simulink model "stage1_robust_loop_model"  (R2026a)
settings: Solver=ode45  StopTime=0.8
undefined symbols (not defined in the file): B, CPR, Ke, Kt, L, R, Ts_disc, V_dc
settings Model: Creator=knavn  LastModifiedBy=knavn

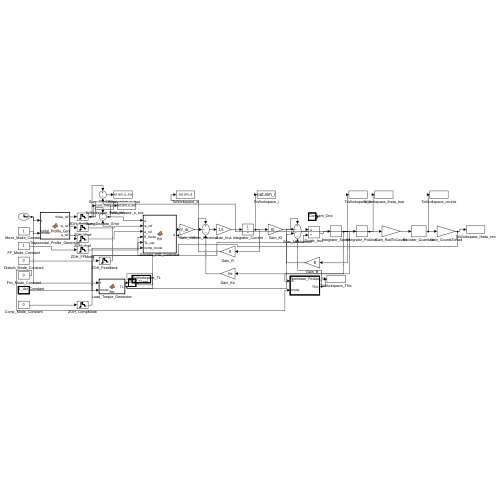
[thumbnail: Simulink's stored preview of the top-level diagram]
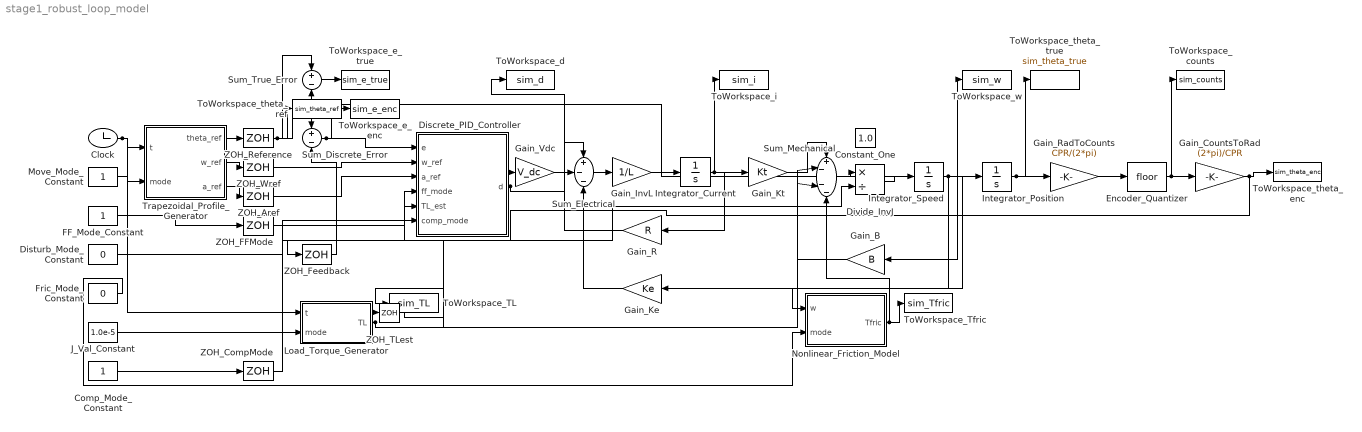
== system stage1_robust_loop_model ==
  Clock : Clock
  Comp_Mode_Constant : Constant
  Constant_One : Constant  Value=1.0
  Discrete_PID_Controller : MATLAB Function  TreatAsAtomicUnit=on
  Disturb_Mode_Constant : Constant  Value=0
  Divide_InvJ : Product  Inputs=*/
  Encoder_Quantizer : Rounding
  FF_Mode_Constant : Constant
  Fric_Mode_Constant : Constant  Value=0
  Gain_B : Gain  Gain=B
  Gain_CountsToRad : Gain  Gain=(2*pi)/CPR
  Gain_InvL : Gain  Gain=1/L
  Gain_Ke : Gain  Gain=Ke
  Gain_Kt : Gain  Gain=Kt
  Gain_R : Gain  Gain=R
  Gain_RadToCounts : Gain  Gain=CPR/(2*pi)
  Gain_Vdc : Gain  Gain=V_dc
  Integrator_Current : Integrator
  Integrator_Position : Integrator
  Integrator_Speed : Integrator
  J_Val_Constant : Constant  Value=1.0e-5
  Load_Torque_Generator : MATLAB Function  TreatAsAtomicUnit=on
  Move_Mode_Constant : Constant
  Nonlinear_Friction_Model : MATLAB Function  TreatAsAtomicUnit=on
  Sum_Discrete_Error : Sum  Inputs=+-
  Sum_Electrical : Sum  Inputs=+--
  Sum_Mechanical : Sum  Inputs=+---
  Sum_True_Error : Sum  Inputs=+-
  ToWorkspace_TL : ToWorkspace  VariableName=sim_TL  SaveFormat=Timeseries  SampleTime=-1
  ToWorkspace_Tfric : ToWorkspace  VariableName=sim_Tfric  SaveFormat=Timeseries  SampleTime=-1
  ToWorkspace_counts : ToWorkspace  VariableName=sim_counts  SaveFormat=Timeseries  SampleTime=-1
  ToWorkspace_d : ToWorkspace  VariableName=sim_d  SaveFormat=Timeseries  SampleTime=-1
  ToWorkspace_e_enc : ToWorkspace  VariableName=sim_e_enc  SaveFormat=Timeseries  SampleTime=-1
  ToWorkspace_e_true : ToWorkspace  VariableName=sim_e_true  SaveFormat=Timeseries  SampleTime=-1
  ToWorkspace_i : ToWorkspace  VariableName=sim_i  SaveFormat=Timeseries  SampleTime=-1
  ToWorkspace_theta_enc : ToWorkspace  VariableName=sim_theta_enc  SaveFormat=Timeseries  SampleTime=-1
  ToWorkspace_theta_ref : ToWorkspace  VariableName=sim_theta_ref  SaveFormat=Timeseries  SampleTime=-1
  ToWorkspace_theta_true : ToWorkspace  VariableName=sim_theta_true  SaveFormat=Timeseries  SampleTime=-1
  ToWorkspace_w : ToWorkspace  VariableName=sim_w  SaveFormat=Timeseries  SampleTime=-1
  Trapezoidal_Profile_Generator : MATLAB Function  TreatAsAtomicUnit=on
  ZOH_Aref : ZeroOrderHold  SampleTime=Ts_disc
  ZOH_CompMode : ZeroOrderHold  SampleTime=Ts_disc
  ZOH_FFMode : ZeroOrderHold  SampleTime=Ts_disc
  ZOH_Feedback : ZeroOrderHold  SampleTime=Ts_disc
  ZOH_Reference : ZeroOrderHold  SampleTime=Ts_disc
  ZOH_TLest : ZeroOrderHold  SampleTime=Ts_disc
  ZOH_Wref : ZeroOrderHold  SampleTime=Ts_disc
  wires:
  Clock/1 -> Trapezoidal_Profile_Generator/1(t), Load_Torque_Generator/1(t)
  Move_Mode_Constant/1 -> Trapezoidal_Profile_Generator/2(mode)
  Trapezoidal_Profile_Generator/1(theta_ref) -> ZOH_Reference/1
  Trapezoidal_Profile_Generator/2(w_ref) -> ZOH_Wref/1
  Trapezoidal_Profile_Generator/3(a_ref) -> ZOH_Aref/1
  ZOH_Reference/1 -> Sum_Discrete_Error/1, Sum_True_Error/1, ToWorkspace_theta_ref/1
  Sum_True_Error/1 -> ToWorkspace_e_true/1
  Sum_Discrete_Error/1 -> Discrete_PID_Controller/1(e), ToWorkspace_e_enc/1
  ZOH_Wref/1 -> Discrete_PID_Controller/2(w_ref)
  ZOH_Aref/1 -> Discrete_PID_Controller/3(a_ref)
  FF_Mode_Constant/1 -> ZOH_FFMode/1
  ZOH_FFMode/1 -> Discrete_PID_Controller/4(ff_mode)
  Disturb_Mode_Constant/1 -> Load_Torque_Generator/2(mode)
  Load_Torque_Generator/1(TL) -> ZOH_TLest/1, Sum_Mechanical/3, ToWorkspace_TL/1
  ZOH_TLest/1 -> Discrete_PID_Controller/5(TL_est)
  Comp_Mode_Constant/1 -> ZOH_CompMode/1
  ZOH_CompMode/1 -> Discrete_PID_Controller/6(comp_mode)
  Discrete_PID_Controller/1(d) -> Gain_Vdc/1, ToWorkspace_d/1
  Gain_Vdc/1 -> Sum_Electrical/1
  Sum_Electrical/1 -> Gain_InvL/1
  Gain_InvL/1 -> Integrator_Current/1
  Integrator_Current/1 -> Gain_R/1, Gain_Kt/1, ToWorkspace_i/1
  Gain_R/1 -> Sum_Electrical/2
  Gain_Kt/1 -> Sum_Mechanical/1
  Sum_Mechanical/1 -> Divide_InvJ/1
  J_Val_Constant/1 -> Divide_InvJ/2
  Divide_InvJ/1 -> Integrator_Speed/1
  Integrator_Speed/1 -> Gain_B/1, Gain_Ke/1, Integrator_Position/1, ToWorkspace_w/1, Nonlinear_Friction_Model/1(w)
  Gain_B/1 -> Sum_Mechanical/2
  Gain_Ke/1 -> Sum_Electrical/3
  Fric_Mode_Constant/1 -> Nonlinear_Friction_Model/2(mode)
  Nonlinear_Friction_Model/1(Tfric) -> Sum_Mechanical/4, ToWorkspace_Tfric/1
  Integrator_Position/1 -> Sum_True_Error/2, ToWorkspace_theta_true/1, Gain_RadToCounts/1
  Gain_RadToCounts/1 -> Encoder_Quantizer/1
  Encoder_Quantizer/1 -> ToWorkspace_counts/1, Gain_CountsToRad/1
  Gain_CountsToRad/1 -> ToWorkspace_theta_enc/1, ZOH_Feedback/1
  ZOH_Feedback/1 -> Sum_Discrete_Error/2

== matlab function stage1_robust_loop_model/Load_Torque_Generator ==
  data: t input; TL output; mode input
function TL = Load_Torque_Generator(t, mode)
if mode == 1 % In-Motion Step at t = 0.200 s
    if t >= 0.200
        TL = 0.010;
    else
        TL = 0.0;
    end
elseif mode == 2 % In-Dwell Pulse at t = 0.600 s (duration 0.150 s)
    if t >= 0.600 && t <= 0.750
        TL = 0.010;
    else
        TL = 0.0;
    end
else
    TL = 0.0;
end
end

== matlab function stage1_robust_loop_model/Trapezoidal_Profile_Generator ==
  data: t input; theta_ref output; mode input; w_ref output; a_ref output
function [theta_ref, w_ref, a_ref] = Trapezoidal_Profile_Generator(t, mode)
a_max = 50.0; w_max = 8.0; step_rad = 90.0 * pi / 180;
t_a = w_max / a_max; theta_a = 0.5 * a_max * t_a^2;
t_c = (step_rad - 2 * theta_a) / w_max; t_f = 2 * t_a + t_c;

if mode == 1
    t_start = 0.050;
    [theta_ref, w_ref, a_ref] = calc_single_move(t, t_start, step_rad, a_max, w_max, t_a, theta_a, t_c, t_f);
else
    [th1, w1, a1] = calc_single_move(t, 0.050, step_rad, a_max, w_max, t_a, theta_a, t_c, t_f);
    [th2, w2, a2] = calc_single_move(t, 0.500, step_rad, a_max, w_max, t_a, theta_a, t_c, t_f);
    [th3, w3, a3] = calc_single_move(t, 0.950, step_rad, a_max, w_max, t_a, theta_a, t_c, t_f);
    theta_ref = th1 + th2 + th3; w_ref = w1 + w2 + w3; a_ref = a1 + a2 + a3;
end
end

function [th, w, a] = calc_single_move(t, t_start, step_rad, a_max, w_max, t_a, theta_a, t_c, t_f)
if t < t_start
    th = 0.0; w = 0.0; a = 0.0;
elseif t < t_start + t_a
    dt = t - t_start;
    th = 0.5 * a_max * dt^2; w = a_max * dt; a = a_max;
elseif t < t_start + t_a + t_c
    dt = t - t_start - t_a;
    th = theta_a + w_max * dt; w = w_max; a = 0.0;
elseif t < t_start + t_f
    dt = t_start + t_f - t;
    th = step_rad - 0.5 * a_max * dt^2; w = a_max * dt; a = -a_max;
else
    th = step_rad; w = 0.0; a = 0.0;
end
end

== matlab function stage1_robust_loop_model/Discrete_PID_Controller ==
  data: e input; d output; w_ref input; a_ref input; ff_mode input; TL_est input; comp_mode input
function d = Discrete_PID_Controller(e, w_ref, a_ref, ff_mode, TL_est, comp_mode)
Kp = 0.50;
Ki = 8.00;
Kd = 0.0000;
N  = 20;
Ts = 0.001;
Kff_v = 0.004175;
Kff_a = 0.00000834;
Kff_L = 0.833333; % Physics Gain: R / (V_dc * Kt) = 0.50 / (12.0 * 0.050)

T_stick = 0.0020;
T_coulomb = 0.0010;
w_s = 0.01;
if abs(w_ref) < 1.0e-6
    Tfric_ref = 0.0;
else
    Tfric_ref = (T_coulomb + (T_stick - T_coulomb) * exp(-(w_ref/w_s)^2)) * tanh(1000 * w_ref);
end

persistent u_i u_d e_prev
if isempty(u_i)
    u_i = 0.0; u_d = 0.0; e_prev = 0.0;
end

u_p = Kp * e;
u_d = (Kd * N * (e - e_prev) + u_d) / (1.0 + N * Ts);
v_i = u_i + Ki * Ts * e;

if ff_mode == 1
    u_ff_kin = Kff_v * w_ref + Kff_a * a_ref;
else
    u_ff_kin = 0.0;
end

if comp_mode == 1 % Active Physics Load & Friction Feedforward Compensation
    u_ff_comp = Kff_L * TL_est + Kff_L * Tfric_ref;
else
    u_ff_comp = 0.0;
end

u_calc = u_p + v_i + u_d + u_ff_kin + u_ff_comp;
if u_calc > 1.0
    d = 1.0;
elseif u_calc < 0.0
    d = 0.0;
else
    d = u_calc;
end

is_sat_high = (u_calc > 1.0) && (e > 0);
is_sat_low  = (u_calc < 0.0) && (e < 0);
if is_sat_high || is_sat_low
    u_i = u_i;
else
    u_i = v_i;
end
e_prev = e;
end

== matlab function stage1_robust_loop_model/Nonlinear_Friction_Model ==
  data: w input; Tfric output; mode input
function Tfric = Nonlinear_Friction_Model(w, mode)
if mode == 0
    Tfric = 0.0;
    return;
end
T_stick = 0.0020;
T_coulomb = 0.0010;
w_s = 0.01;
if abs(w) < 1.0e-6
    Tfric = 0.0;
else
    Tfric = (T_coulomb + (T_stick - T_coulomb) * exp(-(w/w_s)^2)) * tanh(1000 * w);
end
end
